simulink model "array_duty"  (R2014a)
settings: Solver=ode45  StartTime=0.0  StopTime=10.0  RelTol=1e-3
values from neighbouring files (symbols this model uses):
  Tgrid = (1 / Fgrid)    (= 0.0166666666667)    [array_init.m]
undefined symbols (not defined in the file or in its folder): Darray
libraries: simulink x1
settings Model: Creator=Taylor  LastModifiedBy=Taylor

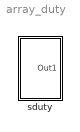
== system array_duty ==
  sduty : Subsystem

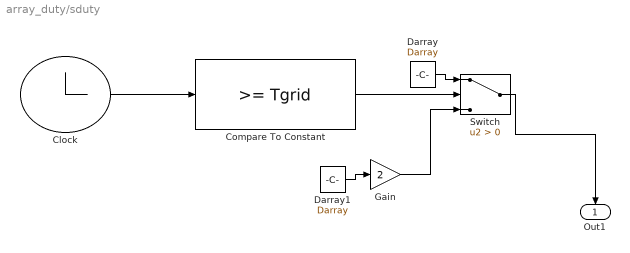
== system array_duty/sduty ==
  Clock : Clock
  Compare To Constant : simulink/Logic and Bit Operations/Compare To Constant  relop=>=  const=Tgrid  OutDataTypeStr=boolean
  Darray : Constant  Value=Darray
  Darray1 : Constant  Value=Darray
  Gain : Gain  Gain=2
  Switch : Switch  Criteria=u2 > Threshold
  Out1 : Outport
  wires:
  Compare To Constant/1 -> Switch/2
  Darray1/1 -> Gain/1
  Darray/1 -> Switch/1
  Switch/1 -> Out1/1
  Gain/1 -> Switch/3
  Clock/1 -> Compare To Constant/1
